simulink model "trabajoControl1"  (R2015a)
settings: Solver=ode45  StartTime=0  StopTime=15  MaxStep=0.01  RelTol=1e-3
model workspace (MAT data in the model file):
  p = [-7.82997288351e-05; 0.181210895977; -0.072497134344; 0.000486358314052; 0.0361674637937]
values from neighbouring files (symbols this model uses):
  Td = 0.0001    [SalidaVelPrimerO.m]    (also in ziegler_nichols.m)
libraries: cstblocks x2, simulink x1
settings Model: Creator=The MathWorks, Inc.  LastModifiedBy=luis_
settings DataIOCC: ExternalInput=[0 0]  InitialState=xstr  LimitDataPoints=off  SaveFormat=StructureWithTime  SaveOutput=off  SaveTime=off  SignalLoggingName=sigsout
settings OptimizationCC: InlineParams=on  InlineInvariantSignals=on  BufferReuse=off  ExpressionDepthLimit=2147483647  InitFltsAndDblsToZero=on  EfficientMapNaN2IntZero=off
settings DebuggingCC: SaveWithParameterizedLinksMsg=none  UnderspecifiedInitializationDetection=Classic  MergeDetectMultiDrivingBlocksExec=none  CheckExecutionContextPreStartOutputMsg=on  CheckExecutionContextRuntimeOutputMsg=on  SignalResolutionControl=TryResolveAllWithWarning  SolverPrmCheckMsg=warning  MultiTaskDSMMsg=warning  FcnCallInpInsideContextMsg=EnableAllAsWarning  StateNameClashWarn=warning
settings GRTTargetCC: TargetFcnLib=ansi_tfl_tmw.mat  CombineOutputUpdateFcns=off  GRTInterface=on

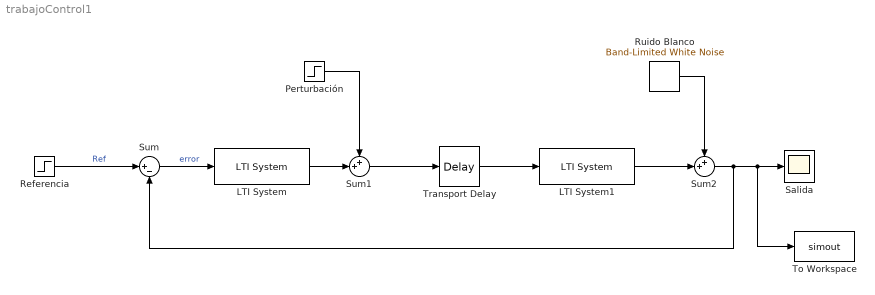
== system trabajoControl1 ==
  LTI System : cstblocks/LTI System  sys=Gclambda  IC=[]
  LTI System1 : cstblocks/LTI System  sys=G1a  IC=[]
  "Perturbación " : Step  After=40  SampleTime=0
  "Referencia " : Step  After=1000  SampleTime=0
  Ruido Blanco : simulink/Sources/Band-Limited White Noise  Cov=[0.1]  Ts=0.001  seed=[23341]
  Salida : Scope
      settings: YMin=-548.9037  YMax=1245.04936
  Sum : Sum  Inputs=|+-
  Sum1 : Sum  Inputs=++|
  Sum2 : Sum  Inputs=++|
  To Workspace : ToWorkspace  VariableName=simout  SaveFormat=Timeseries  SampleTime=-1
  Transport Delay : TransportDelay  DelayTime=Td
  wires:
  "Referencia "/1 -> Sum/1  "Ref"
  Sum1/1 -> Transport Delay/1
  Sum2/1 -> To Workspace/1, Salida/1, Sum/2
  Sum/1 -> LTI System/1  "error"
  LTI System/1 -> Sum1/2
  Transport Delay/1 -> LTI System1/1
  LTI System1/1 -> Sum2/2
  Ruido Blanco/1 -> Sum2/1
  "Perturbación "/1 -> Sum1/1
